simulink model "moto_linearization"  (R2026a)
settings: Solver=VariableStepAuto  StopTime=30
values from neighbouring files (symbols this model uses):
  ft = bs.FrontTire    [bikeSimToMotoParameters.m]
  Gf = Nsh.'*(Oh - B)    [bikeSimToMotoParameters.m]
  Ib = sum(I,3)    [bikeSimToMotoParameters.m]
  If = sum(I,3)    [bikeSimToMotoParameters.m]
  Ift = zeros(3)    [bikeSimToMotoParameters.m]
  Irt = zeros(3)    [bikeSimToMotoParameters.m]
  m = front_bodies(k).m    [bikeSimToMotoParameters.m]
  N = eye(3)    [bikeSimToMotoParameters.m]
  Ob = sum([rear_bodies.O].*[rear_bodies.m],2)/p.mb    [bikeSimToMotoParameters.m]
  p = motoParameters    [bikeSimToMotoParameters.m]    (also in moto_init.m = bikeSimToPrydeV2Parameters(bs,130/3.6); moto_trim_test.m = P{idx_vx}; steadyTurningTrimEqns.m = in3(41,:); steadyTurningTrimJac.m = in3(41,:))
  pf = fpacejka(bs.FrontTire.Pacejka)    [moto_trim_test.m]
  pr = fpacejka(bs.RearTire.Pacejka)    [moto_trim_test.m]
  rt = bs.RearTire    [bikeSimToMotoParameters.m]
  s = linspace(-pi,pi,36)'    [moto_init.m]
  sm = bs.SprungMass    [bikeSimToMotoParameters.m]
  X = zeros(ns,ns,12)    [moto_trim_test.m]
undefined symbols (not defined in the file or in its folder): mb, mh, Rr, Vlow, Y, Z
libraries: sm_lib x60, nesl_utility x51
(part 4 of 5)

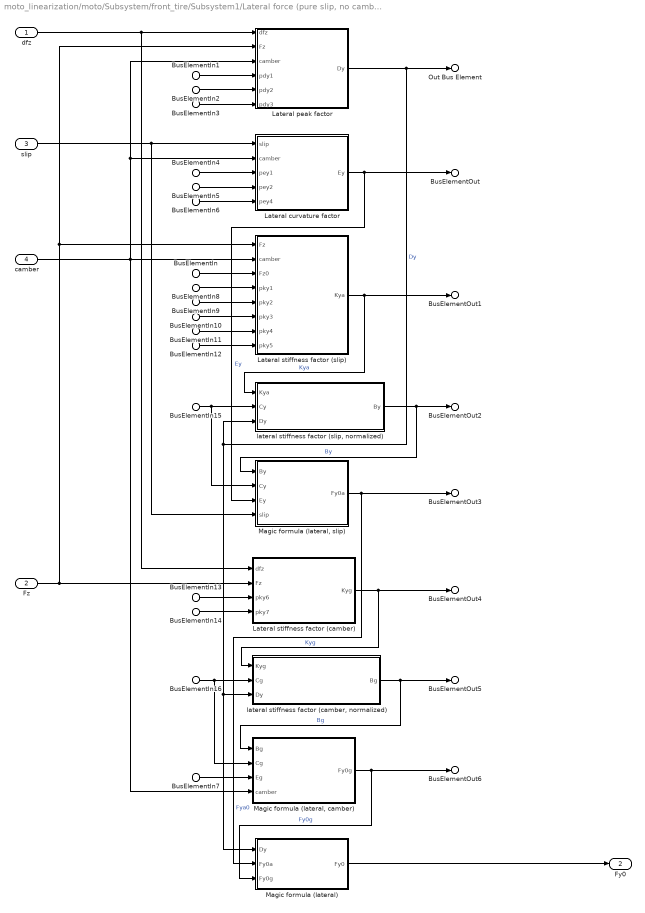
== system moto_linearization/moto/Subsystem/front_tire/Subsystem1/Lateral force (pure slip, no camber) ==
  dfz : Inport
  Fz : Inport  Port=2
  slip : Inport  Port=3
  camber : Inport  Port=4
  BusElementIn : Inport  Port=5  PortName=MF  Element=fz0
  BusElementIn1 : Inport  Port=5  PortName=MF  Element=pdy1
  BusElementIn2 : Inport  Port=5  PortName=MF  Element=pdy2
  BusElementIn3 : Inport  Port=5  PortName=MF  Element=pdy3
  BusElementIn4 : Inport  Port=5  PortName=MF  Element=pey1
  BusElementIn5 : Inport  Port=5  PortName=MF  Element=pey2
  BusElementIn6 : Inport  Port=5  PortName=MF  Element=pey4
  BusElementIn7 : Inport  Port=5  PortName=MF  Element=pey5
  BusElementIn8 : Inport  Port=5  PortName=MF  Element=pky1
  BusElementIn9 : Inport  Port=5  PortName=MF  Element=pky2
  BusElementIn10 : Inport  Port=5  PortName=MF  Element=pky3
  BusElementIn11 : Inport  Port=5  PortName=MF  Element=pky4
  BusElementIn12 : Inport  Port=5  PortName=MF  Element=pky5
  BusElementIn13 : Inport  Port=5  PortName=MF  Element=pky6
  BusElementIn14 : Inport  Port=5  PortName=MF  Element=pky7
  BusElementIn15 : Inport  Port=5  PortName=MF  Element=pcy1
  BusElementIn16 : Inport  Port=5  PortName=MF  Element=pcy2
  Lateral curvature factor : Subsystem
  Lateral peak factor : Subsystem
  Lateral stiffness factor (camber) : Subsystem
  Lateral stiffness factor (slip) : Subsystem
  Magic formula (lateral) : Subsystem
  "Magic formula (lateral, camber)" : Subsystem
  "Magic formula (lateral, slip)" : Subsystem
  "lateral stiffness factor (camber, normalized)" : Subsystem
  "lateral stiffness factor (slip, normalized)" : Subsystem
  Out Bus Element : Outport  PortName=Info  Element=Dy
  BusElementOut : Outport  PortName=Info  Element=Ey
  BusElementOut1 : Outport  PortName=Info  Element=Kya
  BusElementOut2 : Outport  PortName=Info  Element=By
  BusElementOut3 : Outport  PortName=Info  Element=Fy0a
  BusElementOut4 : Outport  PortName=Info  Element=Kyg
  BusElementOut5 : Outport  PortName=Info  Element=Bg
  BusElementOut6 : Outport  PortName=Info  Element=Fy0g
  Fy0 : Outport  Port=2
  wires:
  "Magic formula (lateral, slip)"/1(Fy0a) -> BusElementOut3/1, Magic formula (lateral)/2(Fy0a)  "Fya0"
  "Magic formula (lateral, camber)"/1(Fy0g) -> BusElementOut6/1, Magic formula (lateral)/3(Fy0g)  "Fy0g"
  dfz/1 -> Lateral peak factor/1(dfz), Lateral stiffness factor (camber)/1(dfz)
  BusElementIn/1 -> Lateral stiffness factor (slip)/3(Fz0)
  Fz/1 -> Lateral peak factor/2(Fz), Lateral stiffness factor (slip)/1(Fz), Lateral stiffness factor (camber)/2(Fz)
  BusElementIn3/1 -> Lateral peak factor/6(pdy3)
  BusElementIn12/1 -> Lateral stiffness factor (slip)/8(pky5)
  BusElementIn14/1 -> Lateral stiffness factor (camber)/4(pky7)
  Lateral stiffness factor (camber)/1(Kyg) -> BusElementOut4/1, "lateral stiffness factor (camber, normalized)"/1(Kyg)  "Kyg"
  camber/1 -> "Magic formula (lateral, camber)"/4(camber), Lateral stiffness factor (slip)/2(camber), Lateral peak factor/3(camber), Lateral curvature factor/2(camber)
  "lateral stiffness factor (camber, normalized)"/1(Bg) -> BusElementOut5/1, "Magic formula (lateral, camber)"/1(Bg)  "Bg"
  BusElementIn9/1 -> Lateral stiffness factor (slip)/5(pky2)
  Magic formula (lateral)/1(Fy0) -> Fy0/1
  BusElementIn13/1 -> Lateral stiffness factor (camber)/3(pky6)
  BusElementIn11/1 -> Lateral stiffness factor (slip)/7(pky4)
  BusElementIn15/1 -> "Magic formula (lateral, slip)"/2(Cy), "lateral stiffness factor (slip, normalized)"/2(Cy)
  BusElementIn8/1 -> Lateral stiffness factor (slip)/4(pky1)
  BusElementIn10/1 -> Lateral stiffness factor (slip)/6(pky3)
  BusElementIn4/1 -> Lateral curvature factor/3(pey1)
  slip/1 -> Lateral curvature factor/1(slip), "Magic formula (lateral, slip)"/4(slip)
  BusElementIn6/1 -> Lateral curvature factor/5(pey4)
  BusElementIn16/1 -> "Magic formula (lateral, camber)"/2(Cg), "lateral stiffness factor (camber, normalized)"/2(Cg)
  BusElementIn7/1 -> "Magic formula (lateral, camber)"/3(Eg)
  BusElementIn5/1 -> Lateral curvature factor/4(pey2)
  Lateral peak factor/1(Dy) -> Magic formula (lateral)/1(Dy), "lateral stiffness factor (camber, normalized)"/3(Dy), "lateral stiffness factor (slip, normalized)"/3(Dy), Out Bus Element/1  "Dy"
  "lateral stiffness factor (slip, normalized)"/1(By) -> BusElementOut2/1, "Magic formula (lateral, slip)"/1(By)  "By"
  Lateral stiffness factor (slip)/1(Kya) -> BusElementOut1/1, "lateral stiffness factor (slip, normalized)"/1(Kya)  "Kya"
  BusElementIn2/1 -> Lateral peak factor/5(pdy2)
  BusElementIn1/1 -> Lateral peak factor/4(pdy1)
  Lateral curvature factor/1(Ey) -> BusElementOut/1, "Magic formula (lateral, slip)"/3(Ey)  "Ey"

== system moto_linearization/moto/Subsystem/front_tire/Subsystem1/Longitudinal force (combined slip) ==
  Fx0 : Inport
  slip_ratio : Inport  Port=2
  slip_angle : Inport  Port=3
  BusElementIn : Inport  Port=4  PortName=MF  Element=rbx1
  BusElementIn1 : Inport  Port=4  PortName=MF  Element=rbx2
  BusElementIn2 : Inport  Port=4  PortName=MF  Element=rcx1
  Combined slip : Subsystem
  Longitudinal stiffness factor (combined) : Subsystem
  Fx : Outport
  wires:
  Longitudinal stiffness factor (combined)/1(Bxa) -> Combined slip/1(Bxa)  "Bxa"
  slip_ratio/1 -> Longitudinal stiffness factor (combined)/1(slip_ratio)
  Combined slip/1(Fx) -> Fx/1
  slip_angle/1 -> Combined slip/4(slip_angle)
  Fx0/1 -> Combined slip/3(Fx0)
  BusElementIn2/1 -> Combined slip/2(Cxa)
  BusElementIn1/1 -> Longitudinal stiffness factor (combined)/3(rbx2)
  BusElementIn/1 -> Longitudinal stiffness factor (combined)/2(rbx1)

== system moto_linearization/moto/Subsystem/front_tire/Subsystem1/Longitudinal force (pure slip) ==
  Fz : Inport
  dfz : Inport  Port=2
  slip_ratio : Inport  Port=3
  In Bus Element : Inport  Port=4  PortName=MF  Element=pcx1
  In Bus Element1 : Inport  Port=4  PortName=MF  Element=pdx1
  In Bus Element2 : Inport  Port=4  PortName=MF  Element=pdx2
  In Bus Element3 : Inport  Port=4  PortName=MF  Element=pex1
  In Bus Element4 : Inport  Port=4  PortName=MF  Element=pex2
  In Bus Element5 : Inport  Port=4  PortName=MF  Element=pex3
  In Bus Element6 : Inport  Port=4  PortName=MF  Element=pkx1
  In Bus Element7 : Inport  Port=4  PortName=MF  Element=pkx2
  In Bus Element8 : Inport  Port=4  PortName=MF  Element=pkx3
  Longitudinal curvature factor : Subsystem
  Longitudinal peak factor : Subsystem
  Longitudinal stiffness factor : Subsystem
  Longitudinal stiffness factor (normalized) : Subsystem
  Magic formula (longitudinal) : Subsystem
  Out Bus Element : Outport  PortName=Info  Element=Dx
  BusElementOut : Outport  PortName=Info  Element=Ex
  BusElementOut1 : Outport  PortName=Info  Element=Kx
  BusElementOut2 : Outport  PortName=Info  Element=Bx
  Fx0 : Outport  Port=2
  wires:
  Fz/1 -> Longitudinal peak factor/2(Fz), Longitudinal stiffness factor/2(Fz)
  dfz/1 -> Longitudinal stiffness factor/1(dfz), Longitudinal curvature factor/1(dfz), Longitudinal peak factor/1(dfz)
  Longitudinal stiffness factor (normalized)/1(Bx) -> BusElementOut2/1, Magic formula (longitudinal)/1(Bx)  "Bx"
  slip_ratio/1 -> Longitudinal curvature factor/2(slip_ratio), Magic formula (longitudinal)/5(slip_ratio)
  In Bus Element3/1 -> Longitudinal curvature factor/3(pex1)
  Longitudinal stiffness factor/1(Kx) -> BusElementOut1/1, Longitudinal stiffness factor (normalized)/1(Kx)  "Kx"
  Longitudinal peak factor/1(Dx) -> Out Bus Element/1, Magic formula (longitudinal)/3(Dx), Longitudinal stiffness factor (normalized)/3(Dx)  "Dx"
  In Bus Element/1 -> Magic formula (longitudinal)/2(Cx), Longitudinal stiffness factor (normalized)/2(Cx)
  In Bus Element2/1 -> Longitudinal peak factor/4(pdx2)
  Longitudinal curvature factor/1(Ex) -> BusElementOut/1, Magic formula (longitudinal)/4(Ex)  "Ex"
  Magic formula (longitudinal)/1(Fx0) -> Fx0/1  "Fx0"
  In Bus Element1/1 -> Longitudinal peak factor/3(pdx1)
  In Bus Element5/1 -> Longitudinal curvature factor/5(pex3)
  In Bus Element8/1 -> Longitudinal stiffness factor/5(pkx3)
  In Bus Element6/1 -> Longitudinal stiffness factor/3(pkx1)
  In Bus Element4/1 -> Longitudinal curvature factor/4(pex2)
  In Bus Element7/1 -> Longitudinal stiffness factor/4(pkx2)

== system moto_linearization/moto/Subsystem/front_tire/Subsystem1/MF bus ==
  params : Inport
  Bus Creator1 : BusCreator  Inputs=57
  Demux : Demux  Outputs=57
  MF : Outport
  wires:
  Demux/20 -> Bus Creator1/20  "pey2"
  Demux/56 -> Bus Creator1/56  "mu_ref_x"
  Demux/40 -> Bus Creator1/40  "qcz1"
  Demux/1 -> Bus Creator1/1  "fz0"
  Demux/29 -> Bus Creator1/29  "pky7"
  Demux/17 -> Bus Creator1/17  "pdy2"
  Demux/2 -> Bus Creator1/2  "pcx1"
  Demux/3 -> Bus Creator1/3  "pdx1"
  Demux/33 -> Bus Creator1/33  "rcy1"
  Demux/5 -> Bus Creator1/5  "pex1"
  Demux/57 -> Bus Creator1/57  "mu_ref_y"
  Demux/4 -> Bus Creator1/4  "pdx2"
  params/1 -> Demux/1
  Demux/15 -> Bus Creator1/15  "pcy2"
  Demux/6 -> Bus Creator1/6  "pex2"
  Demux/39 -> Bus Creator1/39  "qbz10"
  Demux/52 -> Bus Creator1/52  "qhz1"
  Demux/22 -> Bus Creator1/22  "pey5"
  Demux/21 -> Bus Creator1/21  "pey4"
  Demux/10 -> Bus Creator1/10  "pkx3"
  Demux/46 -> Bus Creator1/46  "qdz9"
  Demux/42 -> Bus Creator1/42  "qdz2"
  Demux/7 -> Bus Creator1/7  "pex3"
  Demux/11 -> Bus Creator1/11  "rbx1"
  Demux/9 -> Bus Creator1/9  "pkx2"
  Demux/27 -> Bus Creator1/27  "pky5"
  Demux/44 -> Bus Creator1/44  "qdz4"
  Demux/36 -> Bus Creator1/36  "qbz5"
  Bus Creator1/1 -> MF/1  "MF"
  Demux/32 -> Bus Creator1/32  "rby3"
  Demux/8 -> Bus Creator1/8  "pkx1"
  Demux/19 -> Bus Creator1/19  "pey1"
  Demux/14 -> Bus Creator1/14  "pcy1"
  Demux/13 -> Bus Creator1/13  "rcx1"
  Demux/24 -> Bus Creator1/24  "pky2"
  Demux/25 -> Bus Creator1/25  "pky3"
  Demux/16 -> Bus Creator1/16  "pdy1"
  Demux/12 -> Bus Creator1/12  "rbx2"
  Demux/55 -> Bus Creator1/55  "qhz4"
  Demux/18 -> Bus Creator1/18  "pdy3"
  Demux/23 -> Bus Creator1/23  "pky1"
  Demux/26 -> Bus Creator1/26  "pky4"
  Demux/31 -> Bus Creator1/31  "rby2"
  Demux/37 -> Bus Creator1/37  "qbz6"
  Demux/49 -> Bus Creator1/49  "qez1"
  Demux/35 -> Bus Creator1/35  "qbz2"
  Demux/30 -> Bus Creator1/30  "rby1"
  Demux/28 -> Bus Creator1/28  "pky6"
  Demux/34 -> Bus Creator1/34  "qbz1"
  Demux/38 -> Bus Creator1/38  "qbz9"
  Demux/48 -> Bus Creator1/48  "qdz11"
  Demux/41 -> Bus Creator1/41  "qdz1"
  Demux/43 -> Bus Creator1/43  "qdz3"
  Demux/45 -> Bus Creator1/45  "qdz8"
  Demux/47 -> Bus Creator1/47  "qdz10"
  Demux/50 -> Bus Creator1/50  "qez2"
  Demux/51 -> Bus Creator1/51  "qez5"
  Demux/53 -> Bus Creator1/53  "qhz2"
  Demux/54 -> Bus Creator1/54  "qhz3"

== system moto_linearization/moto/Subsystem/front_tire/Subsystem1/Normalized normal force ==
  Fz : Inport
  In Bus Element : Inport  Port=2  PortName=MF  Element=fz0
  Divide : Product  Inputs=*/
  Sum : Sum  Inputs=|+-
  dfz : Outport
  wires:
  Fz/1 -> Sum/1
  In Bus Element/1 -> Sum/2, Divide/2
  Sum/1 -> Divide/1
  Divide/1 -> dfz/1

== system moto_linearization/moto/Subsystem/front_tire/Subsystem1/Residual slip ==
  slip_ratio : Inport
  slip_angle : Inport  Port=2
  SHr : Inport  Port=3
  BusElementIn : Inport  Port=4  PortName=Longitudinal  Element=Kx
  BusElementIn1 : Inport  Port=5  PortName=Lateral  Element=Kya
  Divide : Product  Inputs=*/
  Product1 : Product
  Product2 : Product
  Sign : Signum
  Square : Math  Operator=square
  Square Root : Sqrt
  Square1 : Math  Operator=square
  Sum : Sum  Inputs=|++
  Sum1 : Sum  Inputs=|++
  residual_slip : Outport
  wires:
  slip_angle/1 -> Sum/1
  SHr/1 -> Sum/2
  Sum/1 -> Sign/1, Square/1
  slip_ratio/1 -> Product1/1
  BusElementIn/1 -> Product1/2
  Product1/1 -> Divide/1
  BusElementIn1/1 -> Divide/2
  Divide/1 -> Square1/1
  Square/1 -> Sum1/1
  Square1/1 -> Sum1/2
  Sum1/1 -> Square Root/1
  Sign/1 -> Product2/1
  Square Root/1 -> Product2/2
  Product2/1 -> residual_slip/1

== system moto_linearization/moto/Subsystem/front_tire/Subsystem1/Trail slip ==
  slip_ratio : Inport
  slip_angle : Inport  Port=2
  BusElementIn : Inport  Port=3  PortName=Longitudinal  Element=Kx
  BusElementIn1 : Inport  Port=4  PortName=Lateral  Element=Kya
  Divide : Product  Inputs=*/
  Product1 : Product
  Product2 : Product
  Sign : Signum
  Square : Math  Operator=square
  Square Root : Sqrt
  Square1 : Math  Operator=square
  Sum1 : Sum  Inputs=|++
  trail_slip : Outport
  wires:
  slip_angle/1 -> Sign/1, Square/1
  Sign/1 -> Product2/1
  Square Root/1 -> Product2/2
  Square1/1 -> Sum1/2
  Product1/1 -> Divide/1
  Sum1/1 -> Square Root/1
  Divide/1 -> Square1/1
  Square/1 -> Sum1/1
  Product2/1 -> trail_slip/1
  BusElementIn1/1 -> Divide/2
  BusElementIn/1 -> Product1/2
  slip_ratio/1 -> Product1/1

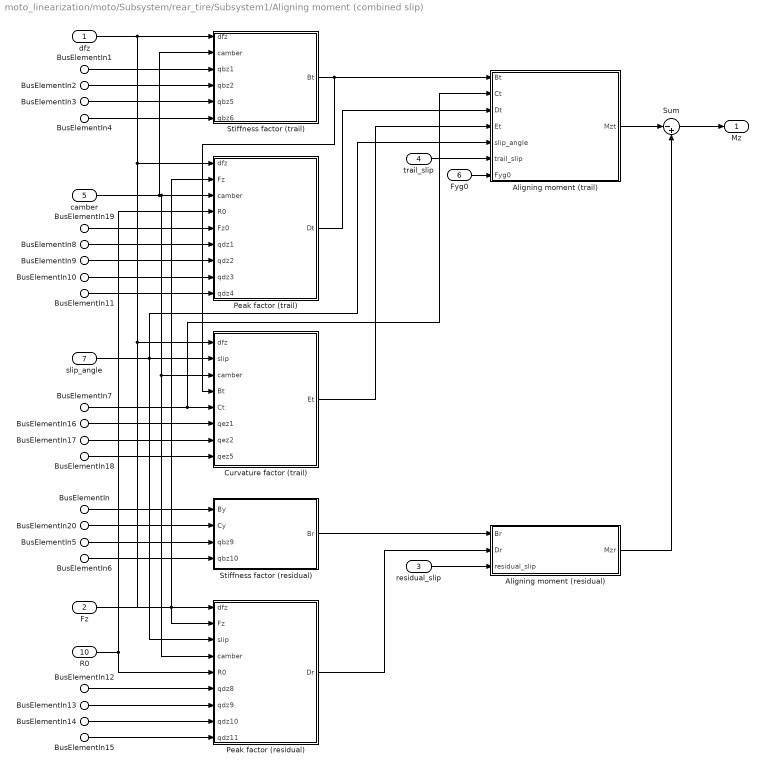
== system moto_linearization/moto/Subsystem/rear_tire/Subsystem1/Aligning moment (combined slip) ==
  dfz : Inport
  Fz : Inport  Port=2
  residual_slip : Inport  Port=3
  trail_slip : Inport  Port=4
  camber : Inport  Port=5
  Fyg0 : Inport  Port=6
  slip_angle : Inport  Port=7
  BusElementIn : Inport  Port=8  PortName=Lateral  Element=By
  BusElementIn1 : Inport  Port=9  PortName=MF  Element=qbz1
  BusElementIn2 : Inport  Port=9  PortName=MF  Element=qbz2
  BusElementIn3 : Inport  Port=9  PortName=MF  Element=qbz5
  BusElementIn4 : Inport  Port=9  PortName=MF  Element=qbz6
  BusElementIn5 : Inport  Port=9  PortName=MF  Element=qbz9
  BusElementIn6 : Inport  Port=9  PortName=MF  Element=qbz10
  BusElementIn7 : Inport  Port=9  PortName=MF  Element=qcz1
  BusElementIn8 : Inport  Port=9  PortName=MF  Element=qdz1
  BusElementIn9 : Inport  Port=9  PortName=MF  Element=qdz2
  BusElementIn10 : Inport  Port=9  PortName=MF  Element=qdz3
  BusElementIn11 : Inport  Port=9  PortName=MF  Element=qdz4
  BusElementIn12 : Inport  Port=9  PortName=MF  Element=qdz8
  BusElementIn13 : Inport  Port=9  PortName=MF  Element=qdz9
  BusElementIn14 : Inport  Port=9  PortName=MF  Element=qdz10
  BusElementIn15 : Inport  Port=9  PortName=MF  Element=qdz11
  BusElementIn16 : Inport  Port=9  PortName=MF  Element=qez1
  BusElementIn17 : Inport  Port=9  PortName=MF  Element=qez2
  BusElementIn18 : Inport  Port=9  PortName=MF  Element=qez5
  BusElementIn19 : Inport  Port=9  PortName=MF  Element=fz0
  BusElementIn20 : Inport  Port=9  PortName=MF  Element=pcy1
  R0 : Inport  Port=10
  Aligning moment (residual) : Subsystem
  Aligning moment (trail) : Subsystem
  Curvature factor (trail) : Subsystem
  Peak factor (residual) : Subsystem
  Peak factor (trail) : Subsystem
  Stiffness factor (residual) : Subsystem
  Stiffness factor (trail) : Subsystem
  Sum : Sum  Inputs=|-+
  Mz : Outport
  wires:
  camber/1 -> Peak factor (residual)/4(camber), Curvature factor (trail)/3(camber), Peak factor (trail)/3(camber), Stiffness factor (trail)/2(camber)
  BusElementIn4/1 -> Stiffness factor (trail)/6(qbz6)
  Peak factor (residual)/1(Dr) -> Aligning moment (residual)/2(Dr)
  slip_angle/1 -> Curvature factor (trail)/2(slip), Aligning moment (trail)/5(slip_angle), Peak factor (residual)/3(slip)
  BusElementIn7/1 -> Aligning moment (trail)/2(Ct), Curvature factor (trail)/5(Ct)
  Aligning moment (residual)/1(Mzr) -> Sum/2
  BusElementIn5/1 -> Stiffness factor (residual)/3(qbz9)
  Aligning moment (trail)/1(Mzt) -> Sum/1
  dfz/1 -> Peak factor (residual)/1(dfz), Curvature factor (trail)/1(dfz), Peak factor (trail)/1(dfz), Stiffness factor (trail)/1(dfz)
  residual_slip/1 -> Aligning moment (residual)/3(residual_slip)
  BusElementIn16/1 -> Curvature factor (trail)/6(qez1)
  Stiffness factor (trail)/1(Bt) -> Aligning moment (trail)/1(Bt), Curvature factor (trail)/4(Bt)
  BusElementIn/1 -> Stiffness factor (residual)/1(By)
  Stiffness factor (residual)/1(Br) -> Aligning moment (residual)/1(Br)
  Fz/1 -> Peak factor (trail)/2(Fz), Peak factor (residual)/2(Fz)
  BusElementIn18/1 -> Curvature factor (trail)/8(qez5)
  R0/1 -> Peak factor (residual)/5(R0), Peak factor (trail)/4(R0)
  Curvature factor (trail)/1(Et) -> Aligning moment (trail)/4(Et)
  BusElementIn19/1 -> Peak factor (trail)/5(Fz0)
  Peak factor (trail)/1(Dt) -> Aligning moment (trail)/3(Dt)
  BusElementIn8/1 -> Peak factor (trail)/6(qdz1)
  BusElementIn14/1 -> Peak factor (residual)/8(qdz10)
  BusElementIn11/1 -> Peak factor (trail)/9(qdz4)
  BusElementIn3/1 -> Stiffness factor (trail)/5(qbz5)
  Sum/1 -> Mz/1
  BusElementIn1/1 -> Stiffness factor (trail)/3(qbz1)
  BusElementIn10/1 -> Peak factor (trail)/8(qdz3)
  trail_slip/1 -> Aligning moment (trail)/6(trail_slip)
  Fyg0/1 -> Aligning moment (trail)/7(Fyg0)
  BusElementIn13/1 -> Peak factor (residual)/7(qdz9)
  BusElementIn15/1 -> Peak factor (residual)/9(qdz11)
  BusElementIn20/1 -> Stiffness factor (residual)/2(Cy)
  BusElementIn6/1 -> Stiffness factor (residual)/4(qbz10)
  BusElementIn9/1 -> Peak factor (trail)/7(qdz2)
  BusElementIn17/1 -> Curvature factor (trail)/7(qez2)
  BusElementIn12/1 -> Peak factor (residual)/6(qdz8)
  BusElementIn2/1 -> Stiffness factor (trail)/4(qbz2)

== system moto_linearization/moto/Subsystem/rear_tire/Subsystem1/Horizontal shift ==
  dfz : Inport
  camber : Inport  Port=2
  BusElementIn : Inport  Port=3  PortName=MF  Element=qhz3
  BusElementIn1 : Inport  Port=3  PortName=MF  Element=qhz4
  Product : Product
  Product1 : Product
  Sum : Sum  Inputs=|++
  SHr : Outport
  wires:
  BusElementIn1/1 -> Product/1
  dfz/1 -> Product/2
  BusElementIn/1 -> Sum/1
  Product/1 -> Sum/2
  Sum/1 -> Product1/1
  camber/1 -> Product1/2
  Product1/1 -> SHr/1

== system moto_linearization/moto/Subsystem/rear_tire/Subsystem1/Lateral force (combined slip) ==
  Fy0 : Inport
  slip_ratio : Inport  Port=2
  slip_angle : Inport  Port=3
  BusElementIn : Inport  Port=4  PortName=MF  Element=rby1
  BusElementIn1 : Inport  Port=4  PortName=MF  Element=rby2
  BusElementIn2 : Inport  Port=4  PortName=MF  Element=rby3
  BusElementIn3 : Inport  Port=4  PortName=MF  Element=rcy1
  Combined slip : Subsystem
  Lateral stiffness factor (combined) : Subsystem
  Fy : Outport
  wires:
  Fy0/1 -> Combined slip/2(Fy0)
  Combined slip/1(Fy) -> Fy/1
  BusElementIn1/1 -> Lateral stiffness factor (combined)/3(rby2)
  BusElementIn3/1 -> Combined slip/4(Cyk)
  slip_ratio/1 -> Combined slip/3(slip_ratio)
  Lateral stiffness factor (combined)/1(Byk) -> Combined slip/1(Byk)
  slip_angle/1 -> Lateral stiffness factor (combined)/1(slip_angle)
  BusElementIn/1 -> Lateral stiffness factor (combined)/2(rby1)
  BusElementIn2/1 -> Lateral stiffness factor (combined)/4(rby3)

== system moto_linearization/moto/Subsystem/rear_tire/Subsystem1/Lateral force (combined slip, no camber) ==
  Fy0 : Inport
  slip_ratio : Inport  Port=2
  slip_angle : Inport  Port=3
  BusElementIn : Inport  Port=4  PortName=MF  Element=rby1
  BusElementIn1 : Inport  Port=4  PortName=MF  Element=rby2
  BusElementIn2 : Inport  Port=4  PortName=MF  Element=rby3
  BusElementIn3 : Inport  Port=4  PortName=MF  Element=rcy1
  Combined slip : Subsystem
  Lateral stiffness factor (combined) : Subsystem
  Fy : Outport
  wires:
  Fy0/1 -> Combined slip/2(Fy0)
  Combined slip/1(Fy) -> Fy/1
  BusElementIn1/1 -> Lateral stiffness factor (combined)/3(rby2)
  BusElementIn3/1 -> Combined slip/4(Cyk)
  slip_ratio/1 -> Combined slip/3(slip_ratio)
  Lateral stiffness factor (combined)/1(Byk) -> Combined slip/1(Byk)
  slip_angle/1 -> Lateral stiffness factor (combined)/1(slip_angle)
  BusElementIn/1 -> Lateral stiffness factor (combined)/2(rby1)
  BusElementIn2/1 -> Lateral stiffness factor (combined)/4(rby3)

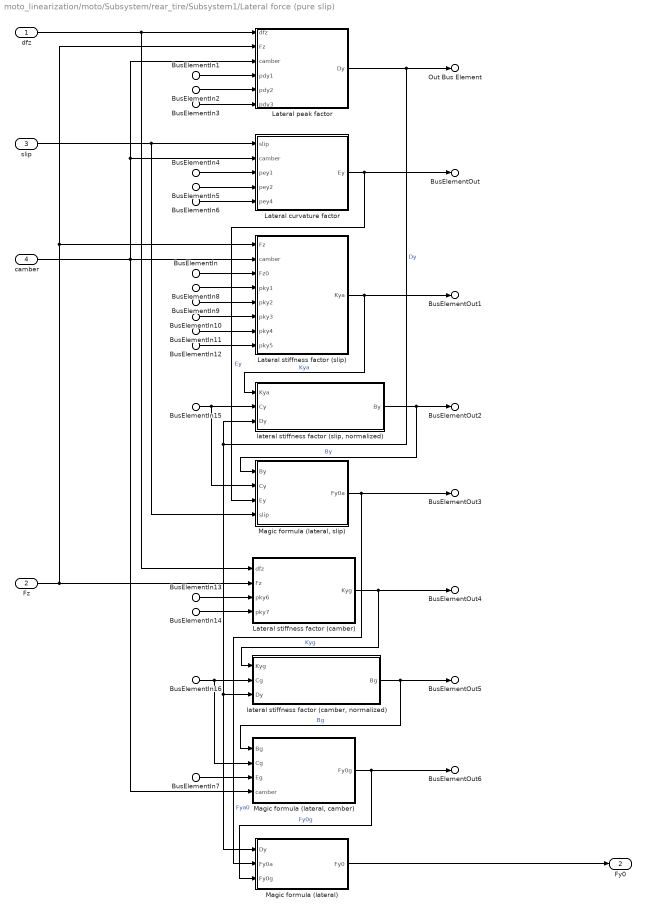
== system moto_linearization/moto/Subsystem/rear_tire/Subsystem1/Lateral force (pure slip) ==
  dfz : Inport
  Fz : Inport  Port=2
  slip : Inport  Port=3
  camber : Inport  Port=4
  BusElementIn : Inport  Port=5  PortName=MF  Element=fz0
  BusElementIn1 : Inport  Port=5  PortName=MF  Element=pdy1
  BusElementIn2 : Inport  Port=5  PortName=MF  Element=pdy2
  BusElementIn3 : Inport  Port=5  PortName=MF  Element=pdy3
  BusElementIn4 : Inport  Port=5  PortName=MF  Element=pey1
  BusElementIn5 : Inport  Port=5  PortName=MF  Element=pey2
  BusElementIn6 : Inport  Port=5  PortName=MF  Element=pey4
  BusElementIn7 : Inport  Port=5  PortName=MF  Element=pey5
  BusElementIn8 : Inport  Port=5  PortName=MF  Element=pky1
  BusElementIn9 : Inport  Port=5  PortName=MF  Element=pky2
  BusElementIn10 : Inport  Port=5  PortName=MF  Element=pky3
  BusElementIn11 : Inport  Port=5  PortName=MF  Element=pky4
  BusElementIn12 : Inport  Port=5  PortName=MF  Element=pky5
  BusElementIn13 : Inport  Port=5  PortName=MF  Element=pky6
  BusElementIn14 : Inport  Port=5  PortName=MF  Element=pky7
  BusElementIn15 : Inport  Port=5  PortName=MF  Element=pcy1
  BusElementIn16 : Inport  Port=5  PortName=MF  Element=pcy2
  Lateral curvature factor : Subsystem
  Lateral peak factor : Subsystem
  Lateral stiffness factor (camber) : Subsystem
  Lateral stiffness factor (slip) : Subsystem
  Magic formula (lateral) : Subsystem
  "Magic formula (lateral, camber)" : Subsystem
  "Magic formula (lateral, slip)" : Subsystem
  "lateral stiffness factor (camber, normalized)" : Subsystem
  "lateral stiffness factor (slip, normalized)" : Subsystem
  Out Bus Element : Outport  PortName=Info  Element=Dy
  BusElementOut : Outport  PortName=Info  Element=Ey
  BusElementOut1 : Outport  PortName=Info  Element=Kya
  BusElementOut2 : Outport  PortName=Info  Element=By
  BusElementOut3 : Outport  PortName=Info  Element=Fy0a
  BusElementOut4 : Outport  PortName=Info  Element=Kyg
  BusElementOut5 : Outport  PortName=Info  Element=Bg
  BusElementOut6 : Outport  PortName=Info  Element=Fy0g
  Fy0 : Outport  Port=2
  wires:
  "Magic formula (lateral, slip)"/1(Fy0a) -> BusElementOut3/1, Magic formula (lateral)/2(Fy0a)  "Fya0"
  "Magic formula (lateral, camber)"/1(Fy0g) -> BusElementOut6/1, Magic formula (lateral)/3(Fy0g)  "Fy0g"
  dfz/1 -> Lateral peak factor/1(dfz), Lateral stiffness factor (camber)/1(dfz)
  BusElementIn/1 -> Lateral stiffness factor (slip)/3(Fz0)
  Fz/1 -> Lateral peak factor/2(Fz), Lateral stiffness factor (slip)/1(Fz), Lateral stiffness factor (camber)/2(Fz)
  BusElementIn3/1 -> Lateral peak factor/6(pdy3)
  BusElementIn12/1 -> Lateral stiffness factor (slip)/8(pky5)
  BusElementIn14/1 -> Lateral stiffness factor (camber)/4(pky7)
  Lateral stiffness factor (camber)/1(Kyg) -> BusElementOut4/1, "lateral stiffness factor (camber, normalized)"/1(Kyg)  "Kyg"
  camber/1 -> "Magic formula (lateral, camber)"/4(camber), Lateral stiffness factor (slip)/2(camber), Lateral peak factor/3(camber), Lateral curvature factor/2(camber)
  "lateral stiffness factor (camber, normalized)"/1(Bg) -> BusElementOut5/1, "Magic formula (lateral, camber)"/1(Bg)  "Bg"
  BusElementIn9/1 -> Lateral stiffness factor (slip)/5(pky2)
  Magic formula (lateral)/1(Fy0) -> Fy0/1
  BusElementIn13/1 -> Lateral stiffness factor (camber)/3(pky6)
  BusElementIn11/1 -> Lateral stiffness factor (slip)/7(pky4)
  BusElementIn15/1 -> "Magic formula (lateral, slip)"/2(Cy), "lateral stiffness factor (slip, normalized)"/2(Cy)
  BusElementIn8/1 -> Lateral stiffness factor (slip)/4(pky1)
  BusElementIn10/1 -> Lateral stiffness factor (slip)/6(pky3)
  BusElementIn4/1 -> Lateral curvature factor/3(pey1)
  slip/1 -> Lateral curvature factor/1(slip), "Magic formula (lateral, slip)"/4(slip)
  BusElementIn6/1 -> Lateral curvature factor/5(pey4)
  BusElementIn16/1 -> "Magic formula (lateral, camber)"/2(Cg), "lateral stiffness factor (camber, normalized)"/2(Cg)
  BusElementIn7/1 -> "Magic formula (lateral, camber)"/3(Eg)
  BusElementIn5/1 -> Lateral curvature factor/4(pey2)
  Lateral peak factor/1(Dy) -> Magic formula (lateral)/1(Dy), "lateral stiffness factor (camber, normalized)"/3(Dy), "lateral stiffness factor (slip, normalized)"/3(Dy), Out Bus Element/1  "Dy"
  "lateral stiffness factor (slip, normalized)"/1(By) -> BusElementOut2/1, "Magic formula (lateral, slip)"/1(By)  "By"
  Lateral stiffness factor (slip)/1(Kya) -> BusElementOut1/1, "lateral stiffness factor (slip, normalized)"/1(Kya)  "Kya"
  BusElementIn2/1 -> Lateral peak factor/5(pdy2)
  BusElementIn1/1 -> Lateral peak factor/4(pdy1)
  Lateral curvature factor/1(Ey) -> BusElementOut/1, "Magic formula (lateral, slip)"/3(Ey)  "Ey"

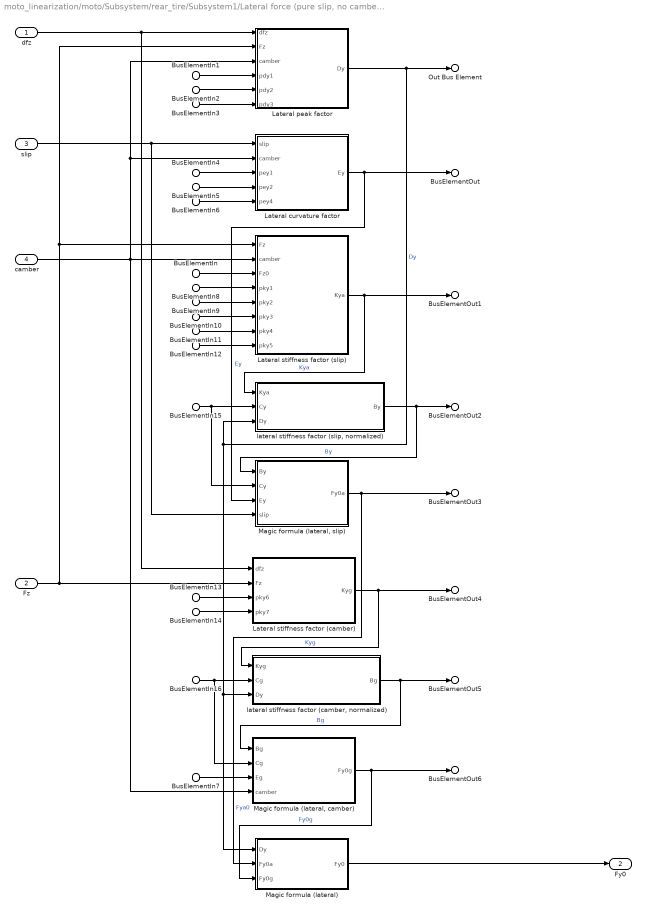
== system moto_linearization/moto/Subsystem/rear_tire/Subsystem1/Lateral force (pure slip, no camber) ==
  dfz : Inport
  Fz : Inport  Port=2
  slip : Inport  Port=3
  camber : Inport  Port=4
  BusElementIn : Inport  Port=5  PortName=MF  Element=fz0
  BusElementIn1 : Inport  Port=5  PortName=MF  Element=pdy1
  BusElementIn2 : Inport  Port=5  PortName=MF  Element=pdy2
  BusElementIn3 : Inport  Port=5  PortName=MF  Element=pdy3
  BusElementIn4 : Inport  Port=5  PortName=MF  Element=pey1
  BusElementIn5 : Inport  Port=5  PortName=MF  Element=pey2
  BusElementIn6 : Inport  Port=5  PortName=MF  Element=pey4
  BusElementIn7 : Inport  Port=5  PortName=MF  Element=pey5
  BusElementIn8 : Inport  Port=5  PortName=MF  Element=pky1
  BusElementIn9 : Inport  Port=5  PortName=MF  Element=pky2
  BusElementIn10 : Inport  Port=5  PortName=MF  Element=pky3
  BusElementIn11 : Inport  Port=5  PortName=MF  Element=pky4
  BusElementIn12 : Inport  Port=5  PortName=MF  Element=pky5
  BusElementIn13 : Inport  Port=5  PortName=MF  Element=pky6
  BusElementIn14 : Inport  Port=5  PortName=MF  Element=pky7
  BusElementIn15 : Inport  Port=5  PortName=MF  Element=pcy1
  BusElementIn16 : Inport  Port=5  PortName=MF  Element=pcy2
  Lateral curvature factor : Subsystem
  Lateral peak factor : Subsystem
  Lateral stiffness factor (camber) : Subsystem
  Lateral stiffness factor (slip) : Subsystem
  Magic formula (lateral) : Subsystem
  "Magic formula (lateral, camber)" : Subsystem
  "Magic formula (lateral, slip)" : Subsystem
  "lateral stiffness factor (camber, normalized)" : Subsystem
  "lateral stiffness factor (slip, normalized)" : Subsystem
  Out Bus Element : Outport  PortName=Info  Element=Dy
  BusElementOut : Outport  PortName=Info  Element=Ey
  BusElementOut1 : Outport  PortName=Info  Element=Kya
  BusElementOut2 : Outport  PortName=Info  Element=By
  BusElementOut3 : Outport  PortName=Info  Element=Fy0a
  BusElementOut4 : Outport  PortName=Info  Element=Kyg
  BusElementOut5 : Outport  PortName=Info  Element=Bg
  BusElementOut6 : Outport  PortName=Info  Element=Fy0g
  Fy0 : Outport  Port=2
  wires:
  "Magic formula (lateral, slip)"/1(Fy0a) -> BusElementOut3/1, Magic formula (lateral)/2(Fy0a)  "Fya0"
  "Magic formula (lateral, camber)"/1(Fy0g) -> BusElementOut6/1, Magic formula (lateral)/3(Fy0g)  "Fy0g"
  dfz/1 -> Lateral peak factor/1(dfz), Lateral stiffness factor (camber)/1(dfz)
  BusElementIn/1 -> Lateral stiffness factor (slip)/3(Fz0)
  Fz/1 -> Lateral peak factor/2(Fz), Lateral stiffness factor (slip)/1(Fz), Lateral stiffness factor (camber)/2(Fz)
  BusElementIn3/1 -> Lateral peak factor/6(pdy3)
  BusElementIn12/1 -> Lateral stiffness factor (slip)/8(pky5)
  BusElementIn14/1 -> Lateral stiffness factor (camber)/4(pky7)
  Lateral stiffness factor (camber)/1(Kyg) -> BusElementOut4/1, "lateral stiffness factor (camber, normalized)"/1(Kyg)  "Kyg"
  camber/1 -> "Magic formula (lateral, camber)"/4(camber), Lateral stiffness factor (slip)/2(camber), Lateral peak factor/3(camber), Lateral curvature factor/2(camber)
  "lateral stiffness factor (camber, normalized)"/1(Bg) -> BusElementOut5/1, "Magic formula (lateral, camber)"/1(Bg)  "Bg"
  BusElementIn9/1 -> Lateral stiffness factor (slip)/5(pky2)
  Magic formula (lateral)/1(Fy0) -> Fy0/1
  BusElementIn13/1 -> Lateral stiffness factor (camber)/3(pky6)
  BusElementIn11/1 -> Lateral stiffness factor (slip)/7(pky4)
  BusElementIn15/1 -> "Magic formula (lateral, slip)"/2(Cy), "lateral stiffness factor (slip, normalized)"/2(Cy)
  BusElementIn8/1 -> Lateral stiffness factor (slip)/4(pky1)
  BusElementIn10/1 -> Lateral stiffness factor (slip)/6(pky3)
  BusElementIn4/1 -> Lateral curvature factor/3(pey1)
  slip/1 -> Lateral curvature factor/1(slip), "Magic formula (lateral, slip)"/4(slip)
  BusElementIn6/1 -> Lateral curvature factor/5(pey4)
  BusElementIn16/1 -> "Magic formula (lateral, camber)"/2(Cg), "lateral stiffness factor (camber, normalized)"/2(Cg)
  BusElementIn7/1 -> "Magic formula (lateral, camber)"/3(Eg)
  BusElementIn5/1 -> Lateral curvature factor/4(pey2)
  Lateral peak factor/1(Dy) -> Magic formula (lateral)/1(Dy), "lateral stiffness factor (camber, normalized)"/3(Dy), "lateral stiffness factor (slip, normalized)"/3(Dy), Out Bus Element/1  "Dy"
  "lateral stiffness factor (slip, normalized)"/1(By) -> BusElementOut2/1, "Magic formula (lateral, slip)"/1(By)  "By"
  Lateral stiffness factor (slip)/1(Kya) -> BusElementOut1/1, "lateral stiffness factor (slip, normalized)"/1(Kya)  "Kya"
  BusElementIn2/1 -> Lateral peak factor/5(pdy2)
  BusElementIn1/1 -> Lateral peak factor/4(pdy1)
  Lateral curvature factor/1(Ey) -> BusElementOut/1, "Magic formula (lateral, slip)"/3(Ey)  "Ey"

== system moto_linearization/moto/Subsystem/rear_tire/Subsystem1/Longitudinal force (combined slip) ==
  Fx0 : Inport
  slip_ratio : Inport  Port=2
  slip_angle : Inport  Port=3
  BusElementIn : Inport  Port=4  PortName=MF  Element=rbx1
  BusElementIn1 : Inport  Port=4  PortName=MF  Element=rbx2
  BusElementIn2 : Inport  Port=4  PortName=MF  Element=rcx1
  Combined slip : Subsystem
  Longitudinal stiffness factor (combined) : Subsystem
  Fx : Outport
  wires:
  Longitudinal stiffness factor (combined)/1(Bxa) -> Combined slip/1(Bxa)  "Bxa"
  slip_ratio/1 -> Longitudinal stiffness factor (combined)/1(slip_ratio)
  Combined slip/1(Fx) -> Fx/1
  slip_angle/1 -> Combined slip/4(slip_angle)
  Fx0/1 -> Combined slip/3(Fx0)
  BusElementIn2/1 -> Combined slip/2(Cxa)
  BusElementIn1/1 -> Longitudinal stiffness factor (combined)/3(rbx2)
  BusElementIn/1 -> Longitudinal stiffness factor (combined)/2(rbx1)

== system moto_linearization/moto/Subsystem/rear_tire/Subsystem1/Longitudinal force (pure slip) ==
  Fz : Inport
  dfz : Inport  Port=2
  slip_ratio : Inport  Port=3
  In Bus Element : Inport  Port=4  PortName=MF  Element=pcx1
  In Bus Element1 : Inport  Port=4  PortName=MF  Element=pdx1
  In Bus Element2 : Inport  Port=4  PortName=MF  Element=pdx2
  In Bus Element3 : Inport  Port=4  PortName=MF  Element=pex1
  In Bus Element4 : Inport  Port=4  PortName=MF  Element=pex2
  In Bus Element5 : Inport  Port=4  PortName=MF  Element=pex3
  In Bus Element6 : Inport  Port=4  PortName=MF  Element=pkx1
  In Bus Element7 : Inport  Port=4  PortName=MF  Element=pkx2
  In Bus Element8 : Inport  Port=4  PortName=MF  Element=pkx3
  Longitudinal curvature factor : Subsystem
  Longitudinal peak factor : Subsystem
  Longitudinal stiffness factor : Subsystem
  Longitudinal stiffness factor (normalized) : Subsystem
  Magic formula (longitudinal) : Subsystem
  Out Bus Element : Outport  PortName=Info  Element=Dx
  BusElementOut : Outport  PortName=Info  Element=Ex
  BusElementOut1 : Outport  PortName=Info  Element=Kx
  BusElementOut2 : Outport  PortName=Info  Element=Bx
  Fx0 : Outport  Port=2
  wires:
  Fz/1 -> Longitudinal peak factor/2(Fz), Longitudinal stiffness factor/2(Fz)
  dfz/1 -> Longitudinal stiffness factor/1(dfz), Longitudinal curvature factor/1(dfz), Longitudinal peak factor/1(dfz)
  Longitudinal stiffness factor (normalized)/1(Bx) -> BusElementOut2/1, Magic formula (longitudinal)/1(Bx)  "Bx"
  slip_ratio/1 -> Longitudinal curvature factor/2(slip_ratio), Magic formula (longitudinal)/5(slip_ratio)
  In Bus Element3/1 -> Longitudinal curvature factor/3(pex1)
  Longitudinal stiffness factor/1(Kx) -> BusElementOut1/1, Longitudinal stiffness factor (normalized)/1(Kx)  "Kx"
  Longitudinal peak factor/1(Dx) -> Out Bus Element/1, Magic formula (longitudinal)/3(Dx), Longitudinal stiffness factor (normalized)/3(Dx)  "Dx"
  In Bus Element/1 -> Magic formula (longitudinal)/2(Cx), Longitudinal stiffness factor (normalized)/2(Cx)
  In Bus Element2/1 -> Longitudinal peak factor/4(pdx2)
  Longitudinal curvature factor/1(Ex) -> BusElementOut/1, Magic formula (longitudinal)/4(Ex)  "Ex"
  Magic formula (longitudinal)/1(Fx0) -> Fx0/1  "Fx0"
  In Bus Element1/1 -> Longitudinal peak factor/3(pdx1)
  In Bus Element5/1 -> Longitudinal curvature factor/5(pex3)
  In Bus Element8/1 -> Longitudinal stiffness factor/5(pkx3)
  In Bus Element6/1 -> Longitudinal stiffness factor/3(pkx1)
  In Bus Element4/1 -> Longitudinal curvature factor/4(pex2)
  In Bus Element7/1 -> Longitudinal stiffness factor/4(pkx2)

== system moto_linearization/moto/Subsystem/rear_tire/Subsystem1/MF bus ==
  params : Inport
  Bus Creator1 : BusCreator  Inputs=57
  Demux : Demux  Outputs=57
  MF : Outport
  wires:
  Demux/20 -> Bus Creator1/20  "pey2"
  Demux/56 -> Bus Creator1/56  "mu_ref_x"
  Demux/40 -> Bus Creator1/40  "qcz1"
  Demux/1 -> Bus Creator1/1  "fz0"
  Demux/29 -> Bus Creator1/29  "pky7"
  Demux/17 -> Bus Creator1/17  "pdy2"
  Demux/2 -> Bus Creator1/2  "pcx1"
  Demux/3 -> Bus Creator1/3  "pdx1"
  Demux/33 -> Bus Creator1/33  "rcy1"
  Demux/5 -> Bus Creator1/5  "pex1"
  Demux/57 -> Bus Creator1/57  "mu_ref_y"
  Demux/4 -> Bus Creator1/4  "pdx2"
  params/1 -> Demux/1
  Demux/15 -> Bus Creator1/15  "pcy2"
  Demux/6 -> Bus Creator1/6  "pex2"
  Demux/39 -> Bus Creator1/39  "qbz10"
  Demux/52 -> Bus Creator1/52  "qhz1"
  Demux/22 -> Bus Creator1/22  "pey5"
  Demux/21 -> Bus Creator1/21  "pey4"
  Demux/10 -> Bus Creator1/10  "pkx3"
  Demux/46 -> Bus Creator1/46  "qdz9"
  Demux/42 -> Bus Creator1/42  "qdz2"
  Demux/7 -> Bus Creator1/7  "pex3"
  Demux/11 -> Bus Creator1/11  "rbx1"
  Demux/9 -> Bus Creator1/9  "pkx2"
  Demux/27 -> Bus Creator1/27  "pky5"
  Demux/44 -> Bus Creator1/44  "qdz4"
  Demux/36 -> Bus Creator1/36  "qbz5"
  Bus Creator1/1 -> MF/1  "MF"
  Demux/32 -> Bus Creator1/32  "rby3"
  Demux/8 -> Bus Creator1/8  "pkx1"
  Demux/19 -> Bus Creator1/19  "pey1"
  Demux/14 -> Bus Creator1/14  "pcy1"
  Demux/13 -> Bus Creator1/13  "rcx1"
  Demux/24 -> Bus Creator1/24  "pky2"
  Demux/25 -> Bus Creator1/25  "pky3"
  Demux/16 -> Bus Creator1/16  "pdy1"
  Demux/12 -> Bus Creator1/12  "rbx2"
  Demux/55 -> Bus Creator1/55  "qhz4"
  Demux/18 -> Bus Creator1/18  "pdy3"
  Demux/23 -> Bus Creator1/23  "pky1"
  Demux/26 -> Bus Creator1/26  "pky4"
  Demux/31 -> Bus Creator1/31  "rby2"
  Demux/37 -> Bus Creator1/37  "qbz6"
  Demux/49 -> Bus Creator1/49  "qez1"
  Demux/35 -> Bus Creator1/35  "qbz2"
  Demux/30 -> Bus Creator1/30  "rby1"
  Demux/28 -> Bus Creator1/28  "pky6"
  Demux/34 -> Bus Creator1/34  "qbz1"
  Demux/38 -> Bus Creator1/38  "qbz9"
  Demux/48 -> Bus Creator1/48  "qdz11"
  Demux/41 -> Bus Creator1/41  "qdz1"
  Demux/43 -> Bus Creator1/43  "qdz3"
  Demux/45 -> Bus Creator1/45  "qdz8"
  Demux/47 -> Bus Creator1/47  "qdz10"
  Demux/50 -> Bus Creator1/50  "qez2"
  Demux/51 -> Bus Creator1/51  "qez5"
  Demux/53 -> Bus Creator1/53  "qhz2"
  Demux/54 -> Bus Creator1/54  "qhz3"

== system moto_linearization/moto/Subsystem/rear_tire/Subsystem1/Normalized normal force ==
  Fz : Inport
  In Bus Element : Inport  Port=2  PortName=MF  Element=fz0
  Divide : Product  Inputs=*/
  Sum : Sum  Inputs=|+-
  dfz : Outport
  wires:
  Fz/1 -> Sum/1
  In Bus Element/1 -> Sum/2, Divide/2
  Sum/1 -> Divide/1
  Divide/1 -> dfz/1

== system moto_linearization/moto/Subsystem/rear_tire/Subsystem1/Residual slip ==
  slip_ratio : Inport
  slip_angle : Inport  Port=2
  SHr : Inport  Port=3
  BusElementIn : Inport  Port=4  PortName=Longitudinal  Element=Kx
  BusElementIn1 : Inport  Port=5  PortName=Lateral  Element=Kya
  Divide : Product  Inputs=*/
  Product1 : Product
  Product2 : Product
  Sign : Signum
  Square : Math  Operator=square
  Square Root : Sqrt
  Square1 : Math  Operator=square
  Sum : Sum  Inputs=|++
  Sum1 : Sum  Inputs=|++
  residual_slip : Outport
  wires:
  slip_angle/1 -> Sum/1
  SHr/1 -> Sum/2
  Sum/1 -> Sign/1, Square/1
  slip_ratio/1 -> Product1/1
  BusElementIn/1 -> Product1/2
  Product1/1 -> Divide/1
  BusElementIn1/1 -> Divide/2
  Divide/1 -> Square1/1
  Square/1 -> Sum1/1
  Square1/1 -> Sum1/2
  Sum1/1 -> Square Root/1
  Sign/1 -> Product2/1
  Square Root/1 -> Product2/2
  Product2/1 -> residual_slip/1

== system moto_linearization/moto/Subsystem/rear_tire/Subsystem1/Trail slip ==
  slip_ratio : Inport
  slip_angle : Inport  Port=2
  BusElementIn : Inport  Port=3  PortName=Longitudinal  Element=Kx
  BusElementIn1 : Inport  Port=4  PortName=Lateral  Element=Kya
  Divide : Product  Inputs=*/
  Product1 : Product
  Product2 : Product
  Sign : Signum
  Square : Math  Operator=square
  Square Root : Sqrt
  Square1 : Math  Operator=square
  Sum1 : Sum  Inputs=|++
  trail_slip : Outport
  wires:
  slip_angle/1 -> Sign/1, Square/1
  Sign/1 -> Product2/1
  Square Root/1 -> Product2/2
  Square1/1 -> Sum1/2
  Product1/1 -> Divide/1
  Sum1/1 -> Square Root/1
  Divide/1 -> Square1/1
  Square/1 -> Sum1/1
  Product2/1 -> trail_slip/1
  BusElementIn1/1 -> Divide/2
  BusElementIn/1 -> Product1/2
  slip_ratio/1 -> Product1/1

== system moto_linearization/moto/Subsystem/front_tire/Subsystem1/Aligning moment (combined slip)/Aligning moment (residual) ==
  Br : Inport
  Dr : Inport  Port=2
  residual_slip : Inport  Port=3
  Atan : Trigonometry  Operator=atan
  Cos : Trigonometry  Operator=cos
  Product : Product
  Product1 : Product
  Mzr : Outport
  wires:
  Br/1 -> Product/1
  residual_slip/1 -> Product/2
  Product/1 -> Atan/1
  Atan/1 -> Cos/1
  Cos/1 -> Product1/1
  Dr/1 -> Product1/2
  Product1/1 -> Mzr/1

== system moto_linearization/moto/Subsystem/front_tire/Subsystem1/Aligning moment (combined slip)/Aligning moment (trail) ==
  Bt : Inport
  Ct : Inport  Port=2
  Dt : Inport  Port=3
  Et : Inport  Port=4
  slip_angle : Inport  Port=5
  trail_slip : Inport  Port=6
  Fyg0 : Inport  Port=7
  Atan : Trigonometry  Operator=atan
  Atan1 : Trigonometry  Operator=atan
  Constant : Constant
  Divide : Product  Inputs=*/
  Product{,1..4} (5 alike) : Product
  Sin : Trigonometry  Operator=cos
  Square : Math  Operator=square
  Square Root : Sqrt
  Sum : Sum  Inputs=|+-
  Sum1 : Sum  Inputs=|+-
  Sum2 : Sum  Inputs=|++
  Mzt : Outport
  wires:
  Dt/1 -> Product3/1
  Sum1/1 -> Atan1/1
  Bt/1 -> Product/1
  Product2/1 -> Sin/1
  Product3/1 -> Divide/1
  Product1/1 -> Sum1/2
  Et/1 -> Product1/1
  trail_slip/1 -> Product/2
  Ct/1 -> Product2/1
  Sum/1 -> Product1/2
  Product/1 -> Sum1/1, Sum/1, Atan/1
  Atan1/1 -> Product2/2
  Atan/1 -> Sum/2
  Sin/1 -> Product3/2
  slip_angle/1 -> Square/1
  Square/1 -> Sum2/1
  Constant/1 -> Sum2/2
  Sum2/1 -> Square Root/1
  Square Root/1 -> Divide/2
  Divide/1 -> Product4/1
  Fyg0/1 -> Product4/2
  Product4/1 -> Mzt/1

== system moto_linearization/moto/Subsystem/front_tire/Subsystem1/Aligning moment (combined slip)/Curvature factor (trail) ==
  dfz : Inport
  slip : Inport  Port=2
  camber : Inport  Port=3
  Bt : Inport  Port=4
  Ct : Inport  Port=5
  qez1 : Inport  Port=6
  qez2 : Inport  Port=7
  qez5 : Inport  Port=8
  Atan : Trigonometry  Operator=atan
  Constant : Constant
  Gain : Gain  Gain=2/pi
  Product : Product  Inputs=3
  Product1 : Product  Inputs=3
  Product2 : Product
  Product3 : Product
  Sum : Sum  Inputs=|++
  Sum1 : Sum  Inputs=|++
  Et : Outport
  wires:
  Bt/1 -> Product/1
  Ct/1 -> Product/2
  slip/1 -> Product/3
  Product/1 -> Atan/1
  Atan/1 -> Gain/1
  Gain/1 -> Product1/1
  camber/1 -> Product1/2
  qez5/1 -> Product1/3
  Product1/1 -> Sum/1
  Constant/1 -> Sum/2
  Sum/1 -> Product2/1
  qez2/1 -> Product3/1
  dfz/1 -> Product3/2
  qez1/1 -> Sum1/1
  Product3/1 -> Sum1/2
  Sum1/1 -> Product2/2
  Product2/1 -> Et/1

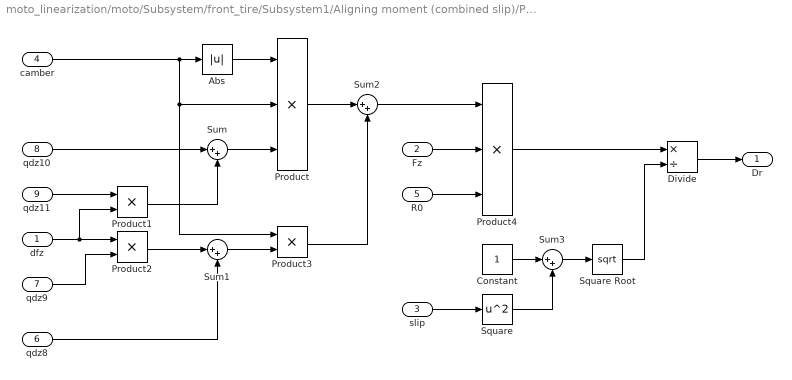
== system moto_linearization/moto/Subsystem/front_tire/Subsystem1/Aligning moment (combined slip)/Peak factor (residual) ==
  dfz : Inport
  Fz : Inport  Port=2
  slip : Inport  Port=3
  camber : Inport  Port=4
  R0 : Inport  Port=5
  qdz8 : Inport  Port=6
  qdz9 : Inport  Port=7
  qdz10 : Inport  Port=8
  qdz11 : Inport  Port=9
  Abs : Abs  SaturateOnIntegerOverflow=off
  Constant : Constant
  Divide : Product  Inputs=*/
  Product : Product  Inputs=3
  Product1 : Product
  Product2 : Product
  Product3 : Product
  Product4 : Product  Inputs=3
  Square : Math  Operator=square
  Square Root : Sqrt
  Sum{,1..3} (4 alike) : Sum  Inputs=|++
  Dr : Outport
  wires:
  camber/1 -> Product3/1, Product/2, Abs/1
  Abs/1 -> Product/1
  qdz11/1 -> Product1/1
  dfz/1 -> Product2/1, Product1/2
  qdz10/1 -> Sum/1
  Product1/1 -> Sum/2
  Sum/1 -> Product/3
  qdz9/1 -> Product2/2
  Product2/1 -> Sum1/1
  qdz8/1 -> Sum1/2
  Sum1/1 -> Product3/2
  Product/1 -> Sum2/1
  Product3/1 -> Sum2/2
  Sum2/1 -> Product4/1
  Fz/1 -> Product4/2
  R0/1 -> Product4/3
  slip/1 -> Square/1
  Square/1 -> Sum3/2
  Constant/1 -> Sum3/1
  Sum3/1 -> Square Root/1
  Product4/1 -> Divide/1
  Square Root/1 -> Divide/2
  Divide/1 -> Dr/1

== system moto_linearization/moto/Subsystem/front_tire/Subsystem1/Aligning moment (combined slip)/Peak factor (trail) ==
  dfz : Inport
  Fz : Inport  Port=2
  camber : Inport  Port=3
  R0 : Inport  Port=4
  Fz0 : Inport  Port=5
  qdz1 : Inport  Port=6
  qdz2 : Inport  Port=7
  qdz3 : Inport  Port=8
  qdz4 : Inport  Port=9
  Abs : Abs  SaturateOnIntegerOverflow=off
  Constant : Constant
  Divide : Product  Inputs=*/
  Product : Product  Inputs=4
  Product1 : Product
  Product2 : Product
  Product3 : Product
  Square : Math  Operator=square
  Sum : Sum  Inputs=|++
  Sum1 : Sum  Inputs=|++
  Sum2 : Sum  Inputs=|++
  Dt : Outport
  wires:
  R0/1 -> Divide/1
  Fz0/1 -> Divide/2
  Divide/1 -> Product/2
  Fz/1 -> Product/1
  dfz/1 -> Product1/2
  qdz2/1 -> Product1/1
  Sum/1 -> Product/3
  Product1/1 -> Sum/2
  qdz1/1 -> Sum/1
  camber/1 -> Square/1, Abs/1
  Abs/1 -> Product2/1
  qdz3/1 -> Product2/2
  Square/1 -> Product3/1
  qdz4/1 -> Product3/2
  Product2/1 -> Sum1/1
  Product3/1 -> Sum1/2
  Sum1/1 -> Sum2/1
  Constant/1 -> Sum2/2
  Sum2/1 -> Product/4
  Product/1 -> Dt/1

== system moto_linearization/moto/Subsystem/front_tire/Subsystem1/Aligning moment (combined slip)/Stiffness factor (residual) ==
  By : Inport
  Cy : Inport  Port=2
  qbz9 : Inport  Port=3
  qbz10 : Inport  Port=4
  Product : Product  Inputs=3
  Sum : Sum  Inputs=|++
  Br : Outport
  wires:
  Cy/1 -> Product/2
  By/1 -> Product/3
  qbz10/1 -> Product/1
  qbz9/1 -> Sum/1
  Product/1 -> Sum/2
  Sum/1 -> Br/1

== system moto_linearization/moto/Subsystem/front_tire/Subsystem1/Aligning moment (combined slip)/Stiffness factor (trail) ==
  dfz : Inport
  camber : Inport  Port=2
  qbz1 : Inport  Port=3
  qbz2 : Inport  Port=4
  qbz5 : Inport  Port=5
  qbz6 : Inport  Port=6
  Abs : Abs  SaturateOnIntegerOverflow=off
  Constant : Constant
  Product{,1..3} (4 alike) : Product
  Square : Math  Operator=square
  Sum : Sum  Inputs=|++
  Sum1 : Sum  Inputs=|++
  Sum2 : Sum  Inputs=|++
  Bt : Outport
  wires:
  qbz2/1 -> Product/1
  dfz/1 -> Product/2
  qbz1/1 -> Sum/1
  Product/1 -> Sum/2
  camber/1 -> Square/1, Abs/1
  Abs/1 -> Product1/1
  qbz5/1 -> Product1/2
  qbz6/1 -> Product2/1
  Square/1 -> Product2/2
  Constant/1 -> Sum1/1
  Product2/1 -> Sum1/2
  Sum1/1 -> Sum2/1
  Product1/1 -> Sum2/2
  Sum2/1 -> Product3/1
  Sum/1 -> Product3/2
  Product3/1 -> Bt/1

== system moto_linearization/moto/Subsystem/front_tire/Subsystem1/Lateral force (combined slip)/Combined slip ==
  Byk : Inport
  Fy0 : Inport  Port=2
  slip_ratio : Inport  Port=3
  Cyk : Inport  Port=4
  Atan : Trigonometry  Operator=atan
  Cos : Trigonometry  Operator=cos
  Product : Product
  Product1 : Product
  Product2 : Product
  Fy : Outport
  wires:
  Byk/1 -> Product/1
  slip_ratio/1 -> Product/2
  Product/1 -> Atan/1
  Atan/1 -> Product1/1
  Cyk/1 -> Product1/2
  Product1/1 -> Cos/1
  Cos/1 -> Product2/1
  Fy0/1 -> Product2/2
  Product2/1 -> Fy/1

== system moto_linearization/moto/Subsystem/front_tire/Subsystem1/Lateral force (combined slip)/Lateral stiffness factor (combined) ==
  slip_angle : Inport
  rby1 : Inport  Port=2
  rby2 : Inport  Port=3
  rby3 : Inport  Port=4
  Atan : Trigonometry  Operator=atan
  Cos : Trigonometry  Operator=cos
  Product : Product
  Product1 : Product
  Sum : Sum  Inputs=|+-
  Byk : Outport
  wires:
  slip_angle/1 -> Sum/1
  rby3/1 -> Sum/2
  Sum/1 -> Product/2
  rby2/1 -> Product/1
  Product/1 -> Atan/1
  Atan/1 -> Cos/1
  Cos/1 -> Product1/2
  rby1/1 -> Product1/1
  Product1/1 -> Byk/1

== system moto_linearization/moto/Subsystem/front_tire/Subsystem1/Lateral force (combined slip, no camber)/Combined slip ==
  Byk : Inport
  Fy0 : Inport  Port=2
  slip_ratio : Inport  Port=3
  Cyk : Inport  Port=4
  Atan : Trigonometry  Operator=atan
  Cos : Trigonometry  Operator=cos
  Product : Product
  Product1 : Product
  Product2 : Product
  Fy : Outport
  wires:
  Byk/1 -> Product/1
  slip_ratio/1 -> Product/2
  Product/1 -> Atan/1
  Atan/1 -> Product1/1
  Cyk/1 -> Product1/2
  Product1/1 -> Cos/1
  Cos/1 -> Product2/1
  Fy0/1 -> Product2/2
  Product2/1 -> Fy/1

== system moto_linearization/moto/Subsystem/front_tire/Subsystem1/Lateral force (combined slip, no camber)/Lateral stiffness factor (combined) ==
  slip_angle : Inport
  rby1 : Inport  Port=2
  rby2 : Inport  Port=3
  rby3 : Inport  Port=4
  Atan : Trigonometry  Operator=atan
  Cos : Trigonometry  Operator=cos
  Product : Product
  Product1 : Product
  Sum : Sum  Inputs=|+-
  Byk : Outport
  wires:
  slip_angle/1 -> Sum/1
  rby3/1 -> Sum/2
  Sum/1 -> Product/2
  rby2/1 -> Product/1
  Product/1 -> Atan/1
  Atan/1 -> Cos/1
  Cos/1 -> Product1/2
  rby1/1 -> Product1/1
  Product1/1 -> Byk/1

== system moto_linearization/moto/Subsystem/front_tire/Subsystem1/Lateral force (pure slip)/Lateral curvature factor ==
  slip : Inport
  camber : Inport  Port=2
  pey1 : Inport  Port=3
  pey2 : Inport  Port=4
  pey4 : Inport  Port=5
  Product : Product  Inputs=3
  Product1 : Product
  Sign : Signum
  Square : Math  Operator=square
  Sum : Sum  Inputs=|++
  Sum1 : Sum  Inputs=|++
  Ey : Outport
  wires:
  slip/1 -> Sign/1
  pey1/1 -> Sum/1
  Sign/1 -> Product/1
  camber/1 -> Square/1, Product/3
  pey4/1 -> Product/2
  Product/1 -> Sum/2
  Sum/1 -> Sum1/1
  Square/1 -> Product1/1
  pey2/1 -> Product1/2
  Product1/1 -> Sum1/2
  Sum1/1 -> Ey/1

== system moto_linearization/moto/Subsystem/front_tire/Subsystem1/Lateral force (pure slip)/Lateral peak factor ==
  dfz : Inport
  Fz : Inport  Port=2
  camber : Inport  Port=3
  pdy1 : Inport  Port=4
  pdy2 : Inport  Port=5
  pdy3 : Inport  Port=6
  Constant : Constant
  Divide : Product  Inputs=*/
  Exp : Math
  Product : Product  Inputs=3
  Product1 : Product
  Product2 : Product
  Square : Math  Operator=square
  Sum : Sum  Inputs=|++
  Dy : Outport
  wires:
  Fz/1 -> Product/1
  pdy1/1 -> Product/2
  pdy2/1 -> Product1/1
  dfz/1 -> Product1/2
  Product1/1 -> Exp/1
  Exp/1 -> Product/3
  camber/1 -> Square/1
  pdy3/1 -> Product2/2
  Square/1 -> Product2/1
  Product/1 -> Divide/1
  Divide/1 -> Dy/1
  Product2/1 -> Sum/1
  Sum/1 -> Divide/2
  Constant/1 -> Sum/2

== system moto_linearization/moto/Subsystem/front_tire/Subsystem1/Lateral force (pure slip)/Lateral stiffness factor (camber) ==
  dfz : Inport
  Fz : Inport  Port=2
  pky6 : Inport  Port=3
  pky7 : Inport  Port=4
  Product : Product
  Product1 : Product
  Sum : Sum  Inputs=|++
  Kyg : Outport
  wires:
  pky7/1 -> Product/1
  dfz/1 -> Product/2
  Product/1 -> Sum/2
  pky6/1 -> Sum/1
  Sum/1 -> Product1/1
  Fz/1 -> Product1/2
  Product1/1 -> Kyg/1

== system moto_linearization/moto/Subsystem/front_tire/Subsystem1/Lateral force (pure slip)/Lateral stiffness factor (slip) ==
  Fz : Inport
  camber : Inport  Port=2
  Fz0 : Inport  Port=3
  pky1 : Inport  Port=4
  pky2 : Inport  Port=5
  pky3 : Inport  Port=6
  pky4 : Inport  Port=7
  pky5 : Inport  Port=8
  Atan : Trigonometry  Operator=atan
  Constant : Constant
  Divide : Product  Inputs=*/
  Divide1 : Product  Inputs=*/
  Product{,1..2,4} (4 alike) : Product
  Product3 : Product  Inputs=3
  Sin : Trigonometry
  Square : Math  Operator=square
  Sum : Sum  Inputs=|++
  Sum1 : Sum  Inputs=|++
  Kya : Outport
  wires:
  camber/1 -> Square/1
  Square/1 -> Product4/1, Product/2
  pky4/1 -> Product/1
  pky3/1 -> Sum/1
  Product/1 -> Sum/2
  Sum/1 -> Product1/2
  Fz0/1 -> Product3/2, Product1/1
  Product1/1 -> Divide/2
  Fz/1 -> Divide/1
  Divide/1 -> Atan/1
  Atan/1 -> Product2/2
  pky2/1 -> Product2/1
  Product2/1 -> Sin/1
  Sin/1 -> Product3/3
  pky1/1 -> Product3/1
  Product3/1 -> Divide1/1
  pky5/1 -> Product4/2
  Product4/1 -> Sum1/1
  Constant/1 -> Sum1/2
  Sum1/1 -> Divide1/2
  Divide1/1 -> Kya/1

== system moto_linearization/moto/Subsystem/front_tire/Subsystem1/Lateral force (pure slip)/Magic formula (lateral) ==
  Dy : Inport
  Fy0a : Inport  Port=2
  Fy0g : Inport  Port=3
  Product : Product
  Sin : Trigonometry
  Sum : Sum  Inputs=|++
  Fy0 : Outport
  wires:
  Fy0a/1 -> Sum/1
  Fy0g/1 -> Sum/2
  Sum/1 -> Sin/1
  Dy/1 -> Product/1
  Sin/1 -> Product/2
  Product/1 -> Fy0/1
